simulink model "mm"  (R2015a)
settings: Solver=ode45  StartTime=0.0  StopTime=26  RelTol=1e-3
values from neighbouring files (symbols this model uses):
  YG = 0.8    [NNPID.m]
undefined symbols (not defined in the file or in its folder): Kp0, Kv0, l, m, Nup, Nuv, X, Y, Z
libraries: sm_lib x10, nesl_utility x5
settings Model: Creator=ANSYSVLAD  LastModifiedBy=ANSYSVLAD
settings SolverCC: ZeroCrossControl=EnableAll  ZeroCrossAlgorithm=Adaptive

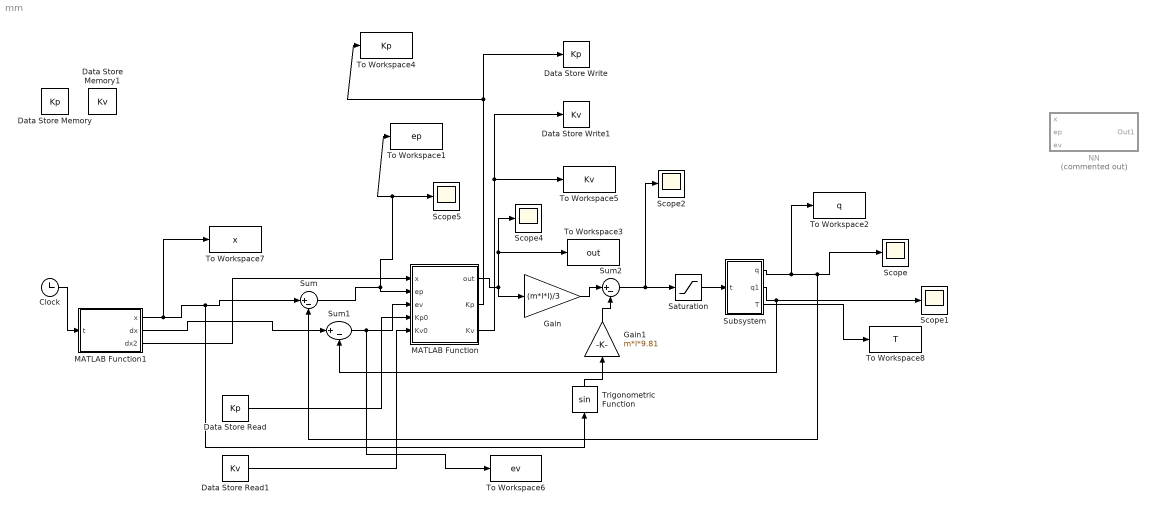
== system mm ==
  Clock : Clock
  Data Store Memory : DataStoreMemory  DataStoreName=Kp  ReadBeforeWriteMsg=warning  WriteAfterWriteMsg=warning  WriteAfterReadMsg=warning  InitialValue=2.5*10^4
  Data Store Memory1 : DataStoreMemory  DataStoreName=Kv  ReadBeforeWriteMsg=warning  WriteAfterWriteMsg=warning  WriteAfterReadMsg=warning  InitialValue=625
  Data Store Read : DataStoreRead  DataStoreName=Kp
  Data Store Read1 : DataStoreRead  DataStoreName=Kv
  Data Store Write : DataStoreWrite  DataStoreName=Kp
  Data Store Write1 : DataStoreWrite  DataStoreName=Kv
  Gain : Gain  Gain=(m*l*l)/3
  Gain1 : Gain  Gain=m*l*9.81
  MATLAB Function : MATLAB Function  TreatAsAtomicUnit=on
  MATLAB Function1 : MATLAB Function  TreatAsAtomicUnit=on
  NN : Subsystem  Commented=on
  Saturation : Saturate  UpperLimit=10  LowerLimit=-10
  Scope{,1..2,4..5} (5 alike) : Scope
      Scope settings: YMin=0.05  YMax=0.275
      Scope2 settings: YMin=0.0003  YMax=0.00105  SaveName=ScopeData2
      Scope4 settings: YMin=4.75  YMax=5.25  SaveName=ScopeData6
      Scope5 settings: YMin=0.00275  YMax=0.0033  SaveName=ScopeData7
  Subsystem : Subsystem
  Sum : Sum  Inputs=|+-
  Sum1 : Sum  Inputs=|+-
  Sum2 : Sum  Inputs=|+-
  To Workspace1 : ToWorkspace  VariableName=ep  SaveFormat=Timeseries  SampleTime=-1
  To Workspace2 : ToWorkspace  VariableName=q  SaveFormat=Timeseries  SampleTime=-1
  To Workspace3 : ToWorkspace  VariableName=out  SaveFormat=Timeseries  SampleTime=-1
  To Workspace4 : ToWorkspace  VariableName=Kp  SaveFormat=Timeseries  SampleTime=-1
  To Workspace5 : ToWorkspace  VariableName=Kv  SaveFormat=Timeseries  SampleTime=-1
  To Workspace6 : ToWorkspace  VariableName=ev  SaveFormat=Timeseries  SampleTime=-1
  To Workspace7 : ToWorkspace  VariableName=x  SaveFormat=Timeseries  SampleTime=-1
  To Workspace8 : ToWorkspace  VariableName=T  SaveFormat=Timeseries  SampleTime=-1
  Trigonometric Function : Trigonometry
  wires:
  MATLAB Function/1(out) -> To Workspace3/1, Scope4/1, Gain/1
  Gain/1 -> Sum2/1
  Sum1/1 -> To Workspace6/1, MATLAB Function/3(ev)
  Sum/1 -> MATLAB Function/2(ep), Scope5/1, To Workspace1/1
  Subsystem/2(q1) -> Sum1/2, Scope1/1
  Sum2/1 -> Saturation/1, Scope2/1
  Gain1/1 -> Sum2/2
  Trigonometric Function/1 -> Gain1/1
  MATLAB Function1/1(x) -> To Workspace7/1, Sum/1, Trigonometric Function/1
  Data Store Read/1 -> MATLAB Function/4(Kp0)
  Data Store Read1/1 -> MATLAB Function/5(Kv0)
  MATLAB Function/3(Kv) -> Data Store Write1/1, To Workspace5/1
  MATLAB Function/2(Kp) -> To Workspace4/1, Data Store Write/1
  Subsystem/1(q) -> To Workspace2/1, Sum/2, Scope/1
  Clock/1 -> MATLAB Function1/1(t)
  MATLAB Function1/3(dx2) -> MATLAB Function/1(x)
  MATLAB Function1/2(dx) -> Sum1/1
  Saturation/1 -> Subsystem/1(t)
  Subsystem/3(T) -> To Workspace8/1

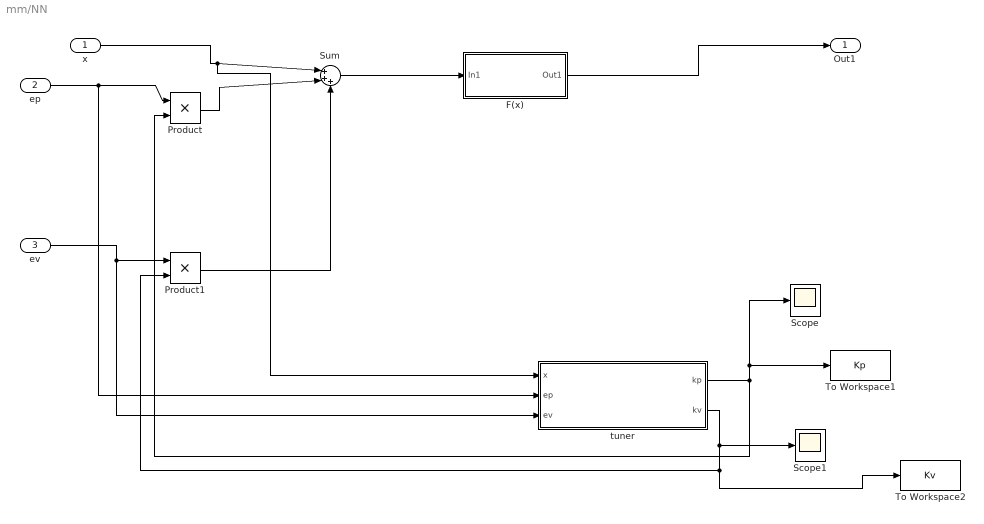
== system mm/NN ==
  x : Inport
  ep : Inport  Port=2
  ev : Inport  Port=3
  F(x) : Subsystem
  Product : Product
  Product1 : Product
  Scope : Scope
      settings: YMin=1e+06  YMax=5.5e+06  SaveName=ScopeData4
  Scope1 : Scope
      settings: YMin=1.03e+07  YMax=1.095e+07  SaveName=ScopeData5
  Sum : Sum  Inputs=|+++
  To Workspace1 : ToWorkspace  VariableName=Kp  SaveFormat=Timeseries  SampleTime=-1
  To Workspace2 : ToWorkspace  VariableName=Kv  SaveFormat=Timeseries  SampleTime=-1
  tuner : Subsystem
  Out1 : Outport
  wires:
  Sum/1 -> F(x)/1(In1)
  F(x)/1(Out1) -> Out1/1
  x/1 -> tuner/1(x), Sum/1
  ep/1 -> Product/1, tuner/2(ep)
  ev/1 -> Product1/1, tuner/3(ev)
  Product/1 -> Sum/2
  Product1/1 -> Sum/3
  tuner/1(kp) -> Scope/1, To Workspace1/1, Product/2
  tuner/2(kv) -> Scope1/1, To Workspace2/1, Product1/2

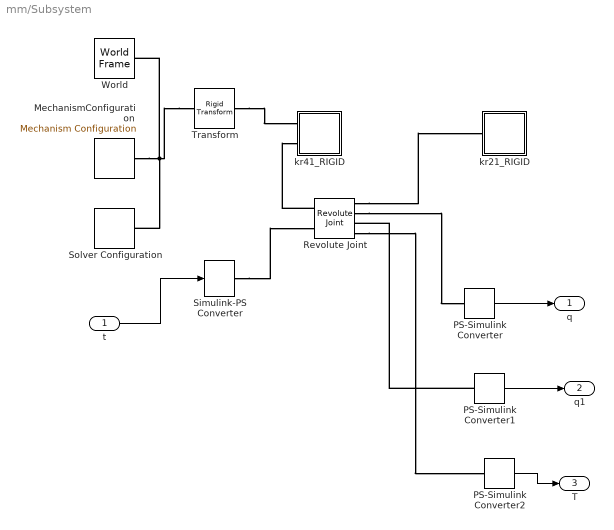
== system mm/Subsystem ==
  t : Inport
  MechanismConfiguration : sm_lib/Utilities/Mechanism Configuration  UniformGravity=Constant  GravityVector=[0 -9.81 0]  GravityUnits=m/s^2  LinearizationDelta=0.001  BlockFunction=simmechanics.library.utilities.mechanism_configuration
  PS-Simulink Converter : nesl_utility/PS-Simulink Converter  PhysicalDomain=network_engine_domain  SubClassName=ps_output  LeftPortType=input  RightPortType=output  PseudoPeriodic=off  Frequencies=[]  Unit=rad  AffineConversion=off
  PS-Simulink Converter1 : nesl_utility/PS-Simulink Converter  PhysicalDomain=network_engine_domain  SubClassName=ps_output  LeftPortType=input  RightPortType=output  PseudoPeriodic=off  Frequencies=[]  Unit=rad/s  AffineConversion=off
  PS-Simulink Converter2 : nesl_utility/PS-Simulink Converter  PhysicalDomain=network_engine_domain  SubClassName=ps_output  LeftPortType=input  RightPortType=output  PseudoPeriodic=off  Frequencies=[]  Unit=N*m  AffineConversion=off
  Revolute Joint : sm_lib/Joints/Revolute Joint  SenseConstraintForce=off  SenseConstraintForceX=off  SenseConstraintForceY=off  SenseConstraintForceZ=off  SenseConstraintTorque=off  SenseConstraintTorqueX=off  SenseConstraintTorqueY=off  SenseConstraintTorqueZ=off  SenseTotalForce=off  SenseTotalForceX=off  SenseTotalForceY=off  SenseTotalForceZ=off  SenseTotalTorque=off  SenseTotalTorqueX=off  SenseTotalTorqueY=off  SenseTotalTorqueZ=off  CompositeWrenchDir=FollowerOnBase  CompositeWrenchFrame=BaseFrame  EquilibriumPosition=0  EquilibriumPositionUnits=deg  SpringStiffness=0  SpringStiffnessUnits=N*m/deg  DampingCoefficient=0  DampingCoefficientUnits=N*m/(deg/s)  TorqueActuationMode=InputTorque  MotionActuationMode=ComputedMotion  SensePosition=on  SenseVelocity=on  SenseAcceleration=off  SenseTorqueForce=on  PositionTargetSpecify=off  PositionTargetPriority=High  PositionTargetValue=0  PositionTargetValueUnits=deg  VelocityTargetSpecify=off  VelocityTargetPriority=High  VelocityTargetValue=0  VelocityTargetValueUnits=deg/s  BlockFunction=simmechanics.library.joints.revolute_joint
  Simulink-PS Converter : nesl_utility/Simulink-PS Converter  PhysicalDomain=network_engine_domain  SubClassName=ps_input  LeftPortType=input  RightPortType=output  PseudoPeriodic=off  Frequencies=[]  NoiseDistribution=none  NoiseParameters=[]  Unit=N*m  AffineConversion=off  InputFiltering=on  SimscapeFilterOrder=1  InputFilterTimeConstant=0.001  UdotUserProvided=1
  Solver Configuration : nesl_utility/Solver Configuration  PhysicalDomain=network_engine_domain  SubClassName=solver  LeftPortType=input  RightPortType=generic  Accelerate=off  Tones=[]  Harmonics=[]  SimulateNoise=off  Profile=off  UseLocalSampling=off  EnableSwitchedLinearOptims=on  FrequencyDomain=off  UseCCode=off  RelTol=0.001  AbsTol=1e-06  MinStep=1e-09  ToWorkspace=off  RevertToSquareIcSolve=off  NumHomotopyIterations=100  DoDC=off  ResidualTolerance=1e-04  UseLocalSolver=off  LocalSolverChoice=NE_BACKWARD_EULER_ADVANCER  LocalSolverSampleTime=1e-6  DoFixedCost=off  MaxNonlinIter=7  MaxModeIter=2  LinearAlgebra=Sparse  DelaysMemoryBudget=1024  AutomaticFiltering=off  FilteringTimeConstant=0.00001
  Transform : sm_lib/Frames and Transforms/Rigid Transform  TranslationMethod=Cartesian  TranslationLengthUnit=mm  TranslationStandardAxis=+Z  TranslationStandardOffset=0  TranslationCartesianOffset=[-2.8703703553210151 -7.1296295233898714 -2.2204460492503131e-15]  TranslationROffset=0  TranslationROffsetUnits=m  TranslationZOffset=0  TranslationZOffsetUnits=m  TranslationThetaOffset=0  TranslationThetaOffsetUnits=deg  RotationMethod=None  RotationAngleUnits=deg  RotationStandardAxis=+Z  RotationAngle=0.0  RotationArbitraryAxis=[0 0 1]  FollAlignAxisA=+X  BaseAlignAxisA=+Y  FollAlignAxisB=+Y  BaseAlignAxisB=+Z  RotationMatrix=[1 0 0; 0 1 0; 0 0 1]  BlockFunction=simmechanics.library.frames_transforms.rigid_transform
  World : sm_lib/Frames and Transforms/World Frame  BlockFunction=simmechanics.library.frames_transforms.world_frame
  kr21_RIGID : Subsystem
  kr41_RIGID : Subsystem
  q : Outport
  q1 : Outport  Port=2
  T : Outport  Port=3
  wires:
  t/1 -> Simulink-PS Converter/1
  PS-Simulink Converter/1 -> q/1
  PS-Simulink Converter1/1 -> q1/1
  PS-Simulink Converter2/1 -> T/1
  connections:
  Transform/LConn1 -- MechanismConfiguration/RConn1 -- Solver Configuration/RConn1 -- World/RConn1
  Revolute Joint/RConn2 -- PS-Simulink Converter/LConn1
  Transform/RConn1 -- kr41_RIGID/LConn1
  Revolute Joint/LConn1 -- kr41_RIGID/LConn2
  Revolute Joint/RConn1 -- kr21_RIGID/LConn1
  PS-Simulink Converter1/LConn1 -- Revolute Joint/RConn3
  Revolute Joint/RConn4 -- PS-Simulink Converter2/LConn1
  Simulink-PS Converter/RConn1 -- Revolute Joint/LConn2

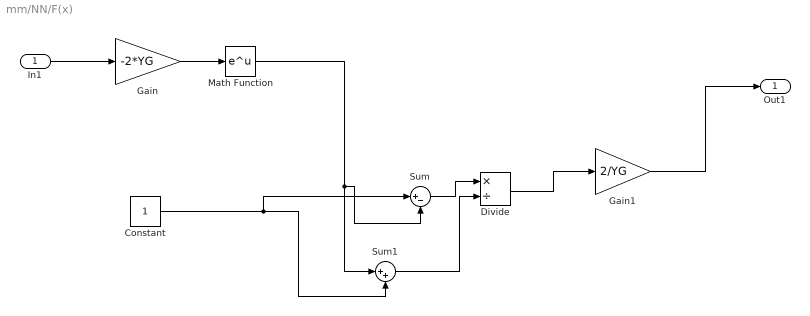
== system mm/NN/F(x) ==
  In1 : Inport
  Constant : Constant
  Divide : Product  Inputs=*/
  Gain : Gain  Gain=-2*YG
  Gain1 : Gain  Gain=2/YG
  Math Function : Math  SaturateOnIntegerOverflow=on
  Sum : Sum  Inputs=|+-
  Sum1 : Sum  Inputs=|++
  Out1 : Outport
  wires:
  In1/1 -> Gain/1
  Gain/1 -> Math Function/1
  Constant/1 -> Sum1/2, Sum/1
  Math Function/1 -> Sum1/1, Sum/2
  Sum/1 -> Divide/1
  Sum1/1 -> Divide/2
  Divide/1 -> Gain1/1
  Gain1/1 -> Out1/1

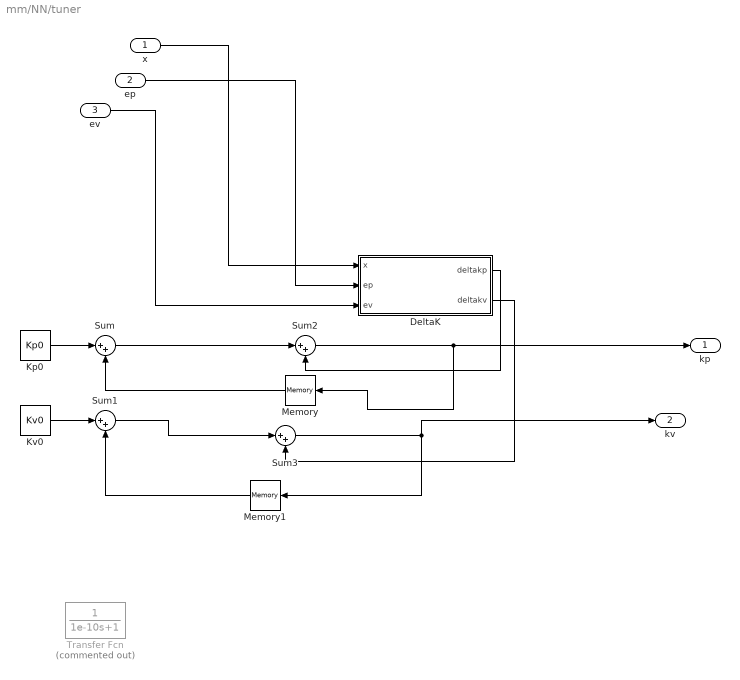
== system mm/NN/tuner ==
  x : Inport
  ep : Inport  Port=2
  ev : Inport  Port=3
  DeltaK : Subsystem
  Kp0 : Constant  Value=Kp0
  Kv0 : Constant  Value=Kv0
  Memory : Memory
  Memory1 : Memory
  Sum{,1..3} (4 alike) : Sum  Inputs=|++
  Transfer Fcn : TransferFcn  Commented=on  Denominator=[1e-10 1]
  kp : Outport
  kv : Outport  Port=2
  wires:
  x/1 -> DeltaK/1(x)
  ep/1 -> DeltaK/2(ep)
  ev/1 -> DeltaK/3(ev)
  Kv0/1 -> Sum1/1
  Kp0/1 -> Sum/1
  Sum/1 -> Sum2/1
  Sum1/1 -> Sum3/1
  Sum3/1 -> Memory1/1, kv/1
  Sum2/1 -> Memory/1, kp/1
  Memory/1 -> Sum/2
  Memory1/1 -> Sum1/2
  DeltaK/1(deltakp) -> Sum2/2
  DeltaK/2("deltakv ") -> Sum3/2

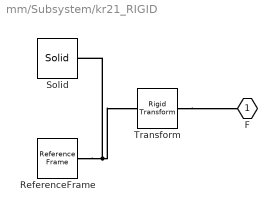
== system mm/Subsystem/kr21_RIGID ==
  ReferenceFrame : sm_lib/Frames and Transforms/Reference Frame  BlockFunction=simmechanics.library.frames_transforms.reference_frame
  Solid : sm_lib/Body Elements/Solid  InertiaType=Custom  Mass=0.30586283305884543  MassUnits=kg  CenterOfMass=[3.6247426023412925e-11 -1.4867689099020885e-14 0]  CenterOfMassUnits=mm  MomentsOfInertia=[1016.7717054457498 83.249573818231923 1018.4578571149564]  MomentsOfInertiaUnits=kg*mm^2  ProductsOfInertia=[-9.0949470177292829e-14 0 -2.728484105320433e-13]  ProductsOfInertiaUnits=kg*mm^2  DensityBased=on  Density=1000  DensityUnits=kg/(m^3)  GraphicType=FromGeometry  MarkerShape=Sphere  MarkerSize=10  MarkerSizeUnits=m  GraphicVisPropType=SimpleVisualProperties  GraphicDiffuseColor=[0.74901960784313726 0.74901960784313726 0.74901960784313726]  GraphicSpecularColor=[0.5 0.5 0.5 1.0]  GraphicAmbientColor=[0.15 0.15 0.15 1.0]  GraphicEmissiveColor=[0.0 0.0 0.0 1.0]  GraphicShininess=75  GraphicOpacity=1  GeometryShape=FromFile  RectangleSize=[1 1]  RectangleSizeUnits=m  BrickDimensions=[1 1 1]  BrickDimensionUnits=m  CylinderRadius=1  CylinderRadiusUnits=m  CylinderLength=1  CylinderLengthUnits=m  SphereRadius=1  SphereRadiusUnits=m  EllipsoidRadii=[1 1 1]  EllipsoidRadiiUnits=m  ExtrusionCrossSection=[1 1; -1 1; -1 -1; 1 -1]  ExtrusionCrossSectionUnits=m  ExtrusionLength=1  ExtrusionLengthUnits=m  PolygonNumSides=3  PolygonOuterRadius=1  PolygonOuterRadiusUnits=m  ExtGeomFileType=STL  ExtGeomFileName=kr2_ipt_1247a2ad.STL  ExtGeomFileUnits=mm  RevolutionCrossSection=[1 1; 1 -1; 2 -1; 2 1]  RevolutionCrossSectionUnits=m  RevolutionExtent=Full  RevolutionAngle=180  RevolutionAngleUnits=deg  BlockFunction=simmechanics.library.body_elements.solid
  Transform : sm_lib/Frames and Transforms/Rigid Transform  TranslationMethod=Cartesian  TranslationLengthUnit=mm  TranslationStandardAxis=+Z  TranslationStandardOffset=0  TranslationCartesianOffset=[1.1102230246251565e-15 -80.000000000000213 0]  TranslationROffset=0  TranslationROffsetUnits=m  TranslationZOffset=0  TranslationZOffsetUnits=m  TranslationThetaOffset=0  TranslationThetaOffsetUnits=deg  RotationMethod=ArbitraryAxis  RotationAngleUnits=rad  RotationStandardAxis=+Z  RotationAngle=0  RotationArbitraryAxis=[0 0 0]  FollAlignAxisA=+X  BaseAlignAxisA=+Y  FollAlignAxisB=+Y  BaseAlignAxisB=+Z  RotationMatrix=[1 0 0; 0 1 0; 0 0 1]  BlockFunction=simmechanics.library.frames_transforms.rigid_transform
  F : PMIOPort  Port=1  Side=Left
  connections:
  Solid/RConn1 -- ReferenceFrame/RConn1 -- Transform/LConn1
  Transform/RConn1 -- F/RConn1

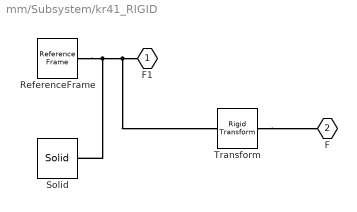
== system mm/Subsystem/kr41_RIGID ==
  ReferenceFrame : sm_lib/Frames and Transforms/Reference Frame  BlockFunction=simmechanics.library.frames_transforms.reference_frame
  Solid : sm_lib/Body Elements/Solid  InertiaType=Custom  Mass=0.13693141652942267  MassUnits=kg  CenterOfMass=[4.0482822334017741e-11 0 0]  CenterOfMassUnits=mm  MomentsOfInertia=[61.358120268124317 61.358120242449267 86.201196102727565]  MomentsOfInertiaUnits=kg*mm^2  ProductsOfInertia=[0 0 0]  ProductsOfInertiaUnits=kg*mm^2  DensityBased=on  Density=1000  DensityUnits=kg/(m^3)  GraphicType=FromGeometry  MarkerShape=Sphere  MarkerSize=10  MarkerSizeUnits=m  GraphicVisPropType=SimpleVisualProperties  GraphicDiffuseColor=[0.74901960784313726 0.74901960784313726 0.74901960784313726]  GraphicSpecularColor=[0.5 0.5 0.5 1.0]  GraphicAmbientColor=[0.15 0.15 0.15 1.0]  GraphicEmissiveColor=[0.0 0.0 0.0 1.0]  GraphicShininess=75  GraphicOpacity=1  GeometryShape=FromFile  RectangleSize=[1 1]  RectangleSizeUnits=m  BrickDimensions=[1 1 1]  BrickDimensionUnits=m  CylinderRadius=1  CylinderRadiusUnits=m  CylinderLength=1  CylinderLengthUnits=m  SphereRadius=1  SphereRadiusUnits=m  EllipsoidRadii=[1 1 1]  EllipsoidRadiiUnits=m  ExtrusionCrossSection=[1 1; -1 1; -1 -1; 1 -1]  ExtrusionCrossSectionUnits=m  ExtrusionLength=1  ExtrusionLengthUnits=m  PolygonNumSides=3  PolygonOuterRadius=1  PolygonOuterRadiusUnits=m  ExtGeomFileType=STL  ExtGeomFileName=kr4_ipt_3bad97a.STL  ExtGeomFileUnits=mm  RevolutionCrossSection=[1 1; 1 -1; 2 -1; 2 1]  RevolutionCrossSectionUnits=m  RevolutionExtent=Full  RevolutionAngle=180  RevolutionAngleUnits=deg  BlockFunction=simmechanics.library.body_elements.solid
  Transform : sm_lib/Frames and Transforms/Rigid Transform  TranslationMethod=Cartesian  TranslationLengthUnit=mm  TranslationStandardAxis=+Z  TranslationStandardOffset=0  TranslationCartesianOffset=[-1.1857181902996672e-13 -3.4994229736184934e-13 40]  TranslationROffset=0  TranslationROffsetUnits=m  TranslationZOffset=0  TranslationZOffsetUnits=m  TranslationThetaOffset=0  TranslationThetaOffsetUnits=deg  RotationMethod=ArbitraryAxis  RotationAngleUnits=rad  RotationStandardAxis=+Z  RotationAngle=0.12768539142570112  RotationArbitraryAxis=[-0 -0 -1]  FollAlignAxisA=+X  BaseAlignAxisA=+Y  FollAlignAxisB=+Y  BaseAlignAxisB=+Z  RotationMatrix=[1 0 0; 0 1 0; 0 0 1]  BlockFunction=simmechanics.library.frames_transforms.rigid_transform
  F1 : PMIOPort  Port=1  Side=Left
  F : PMIOPort  Port=2  Side=Left
  connections:
  Solid/RConn1 -- ReferenceFrame/RConn1 -- Transform/LConn1 -- F1/RConn1
  Transform/RConn1 -- F/RConn1

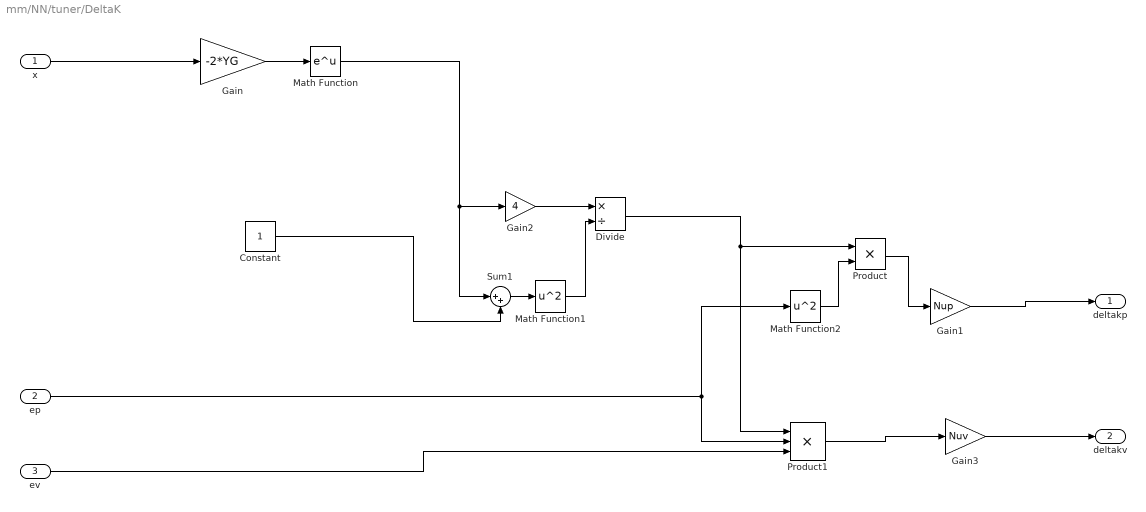
== system mm/NN/tuner/DeltaK ==
  x : Inport
  ep : Inport  Port=2
  ev : Inport  Port=3
  Constant : Constant
  Divide : Product  Inputs=*/
  Gain : Gain  Gain=-2*YG
  Gain1 : Gain  Gain=Nup
  Gain2 : Gain  Gain=4
  Gain3 : Gain  Gain=Nuv
  Math Function : Math  OutputSignalType=real  SaturateOnIntegerOverflow=on
  Math Function1 : Math  Operator=square  OutputSignalType=real  SaturateOnIntegerOverflow=on
  Math Function2 : Math  Operator=square  OutputSignalType=real  SaturateOnIntegerOverflow=on
  Product : Product
  Product1 : Product  Inputs=3
  Sum1 : Sum  Inputs=|++
  deltakp : Outport
  "deltakv " : Outport  Port=2
  wires:
  ev/1 -> Product1/3
  Gain1/1 -> deltakp/1
  Product1/1 -> Gain3/1
  Sum1/1 -> Math Function1/1
  Divide/1 -> Product1/1, Product/1
  Gain2/1 -> Divide/1
  Gain/1 -> Math Function/1
  Math Function2/1 -> Product/2
  Gain3/1 -> "deltakv "/1
  Constant/1 -> Sum1/2
  x/1 -> Gain/1
  Math Function/1 -> Gain2/1, Sum1/1
  ep/1 -> Product1/2, Math Function2/1
  Math Function1/1 -> Divide/2
  Product/1 -> Gain1/1

== matlab function mm/MATLAB Function1 ==
  data: t input; x output; dx output; dx2 output
function [x,dx,dx2] = fcn(t)
dx = cos(t);
dx2 = -sin(t);
x = sin(t);

== matlab function mm/MATLAB Function ==
  data: x input; out output; ep input; ev input; Kp0 input; Kv0 input; Kp output; Kv output
function [out,Kp,Kv] = NNPID(x,ep,ev, Kp0, Kv0)
nup = 7*10^4;
nuv = 100;
YG = 0.8;
deltaKp = nup * ep^2 * ((4*exp(-2*x*YG))/(1 + exp(-2*x*YG))^2);
deltaKv = nuv * ep * ev * ((4*exp(-2*x*YG))/(1 + exp(-2*x*YG))^2);
out = x + Kp0*ep + Kv0*ev;
Kp = Kp0 + deltaKp;
Kv = Kv0 + deltaKv;
